simulink model "sbsb_srs_edit_7"  (R2023b)
settings: Solver=FixedStepDiscrete  StartTime=0.0  StopTime=100  FixedStep=0.001  RelTol=1e-3
libraries: Solver_SF x1
settings Model: DataTypeOverride=Double  MinMaxOverflowLogging=ForceOff  Creator=황수빈  LastModifiedBy=황수빈

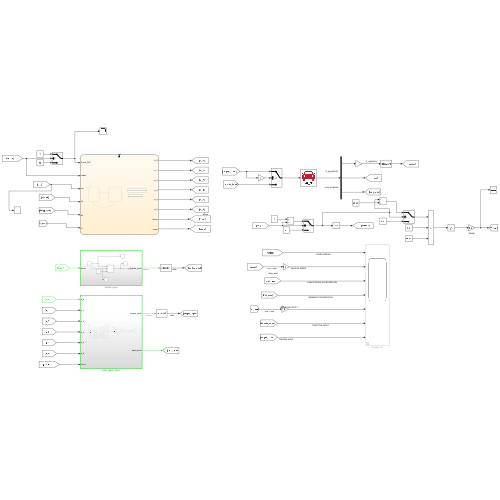
[thumbnail: Simulink's stored preview of the top-level diagram]
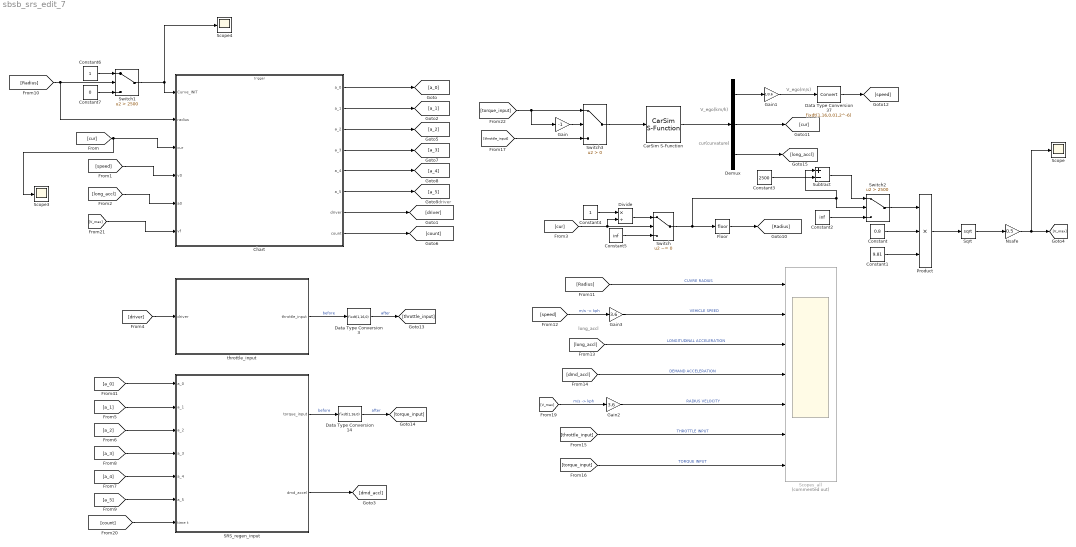
== system sbsb_srs_edit_7 ==
  note: driver
  note: long_accl
  note: V_ego(km/h)
  note: V_ego(m/s)
  note: cur(curvature)
  CarSim S-Function : Solver_SF/CarSim S-Function  Priority=1  SIMFILE=simfile.sim  Run_RTs=off  vs_state_ind=Run  StopMode_ind=Vehicle Model
  Chart : Stateflow chart  TreatAsAtomicUnit=on
  Constant : Constant  Value=0.8
  Constant1 : Constant  Value=9.81
  Constant2 : Constant  Value=inf
  Constant3 : Constant  Value=2500
  Constant4 : Constant
  Constant5 : Constant  Value=inf
  Constant6 : Constant
  Constant7 : Constant  Value=0
  Data Type Conversion14 : DataTypeConversion  OutDataTypeStr=fixdt(1,16,0)  RndMeth=Nearest  SaturateOnIntegerOverflow=off
  Data Type Conversion3 : DataTypeConversion  OutDataTypeStr=fixdt(1,16,0)  RndMeth=Nearest  SaturateOnIntegerOverflow=off
  Data Type Conversion37 : DataTypeConversion  OutDataTypeStr=fixdt(1,16,0.01,2^-6)  RndMeth=Simplest  SaturateOnIntegerOverflow=off
  Demux : Demux  Outputs=3
  Divide : Product  Inputs=*/
  Floor : Rounding
  Gain : Gain  Gain=-1
  Gain1 : Gain  Gain=1/3.6
  Gain2 : Gain  Gain=3.6
  Gain3 : Gain  Gain=3.6
  Nsafe : Gain  Gain=0.5
  Product : Product  Inputs=3
  SRS_regen_input : Subsystem  TreatAsAtomicUnit=on
  Scope : Scope
  Scope3 : Scope
  Scope4 : Scope
  Scopes_all : Scope  Commented=on  NumInputPorts=7
  Sqrt : Sqrt
  Subtract : Sum  Inputs=+-
  Switch : Switch  Criteria=u2 ~= 0  SaturateOnIntegerOverflow=off  InputSameDT=off
  Switch1 : Switch  Criteria=u2 > Threshold  Threshold=2500  SaturateOnIntegerOverflow=off  InputSameDT=off
  Switch2 : Switch  Criteria=u2 > Threshold  Threshold=2500  SaturateOnIntegerOverflow=off  InputSameDT=off
  Switch3 : Switch  Criteria=u2 > Threshold  SaturateOnIntegerOverflow=off  InputSameDT=off
  throttle_input : Subsystem  TreatAsAtomicUnit=on  SystemSampleTime=0.01
  wires:
  Chart/7(driver) -> [driver]
  [cur] -> Scope3/1, Chart/3(cur)
  [speed] -> Chart/4(v0)
  [long_accl] -> Chart/5(a0)
  Chart/1(a_0) -> [a_0]
  Chart/2(a_1) -> [a_1]
  Chart/3(a_2) -> [a_2]
  Chart/4(a_3) -> [a_3]
  Chart/5(a_4) -> [a_4]
  Chart/6(a_5) -> [a_5]
  Switch/1 -> Floor/1, Subtract/1, Switch2/2
  [cur] -> Switch/2, Divide/2
  Constant5/1 -> Switch/3
  Constant4/1 -> Divide/1
  Divide/1 -> Switch/1
  Gain1/1 -> Data Type Conversion37/1
  Demux/1 -> Gain1/1
  Demux/2 -> [cur]
  Data Type Conversion37/1 -> [speed]
  CarSim S-Function/1 -> Demux/1
  [driver] -> throttle_input/1(driver)
  Data Type Conversion3/1 -> [throttle_input]  "after"
  throttle_input/1(throttle_input) -> Data Type Conversion3/1  "before"
  SRS_regen_input/1(torque_input) -> Data Type Conversion14/1  "before"
  [a_2] -> SRS_regen_input/3(a_2)
  Data Type Conversion14/1 -> [torque_input]  "after"
  [a_0] -> SRS_regen_input/1(a_0)
  [a_3] -> SRS_regen_input/4(a_3)
  [a_5] -> SRS_regen_input/6(a_5)
  [Radius] -> Chart/2(radius), Switch1/2
  Constant6/1 -> Switch1/1
  Switch1/1 -> Scope4/1, Chart/1(Curve_INIT)
  Constant7/1 -> Switch1/3
  Demux/3 -> [long_accl]
  [Radius] -> Scopes_all/1  "CUVRE RADIUS"
  [speed] -> Gain3/1  "m/s -> kph"
  [long_accl] -> Scopes_all/3  "LONGITUDINAL ACCELERATION"
  [dmd_accl] -> Scopes_all/4  "DEMAND ACCELERATION"
  [V_max] -> Gain2/1  "m/s -> kph"
  [throttle_input] -> Scopes_all/6  "THROTTLE INPUT"
  SRS_regen_input/2(dmd_accel) -> [dmd_accl]
  Gain2/1 -> Scopes_all/5  "RADIUS VELOCITY"
  [a_1] -> SRS_regen_input/2(a_1)
  [a_4] -> SRS_regen_input/5(a_4)
  Chart/8(count) -> [count]
  [count] -> SRS_regen_input/7(time t)
  Sqrt/1 -> Nsafe/1
  Switch2/1 -> Product/1
  Constant/1 -> Product/2
  Constant1/1 -> Product/3
  Product/1 -> Sqrt/1
  Constant2/1 -> Switch2/3
  Nsafe/1 -> Scope/1, [V_max]
  [V_max] -> Chart/6(vf)
  Floor/1 -> [Radius]
  Switch3/1 -> CarSim S-Function/1
  [torque_input] -> Gain/1, Switch3/1
  [throttle_input] -> Switch3/3
  Gain/1 -> Switch3/2
  Constant3/1 -> Subtract/2
  Subtract/1 -> Switch2/1
  Gain3/1 -> Scopes_all/2  "VEHICLE SPEED"
  [torque_input] -> Scopes_all/7  "TORQUE INPUT"

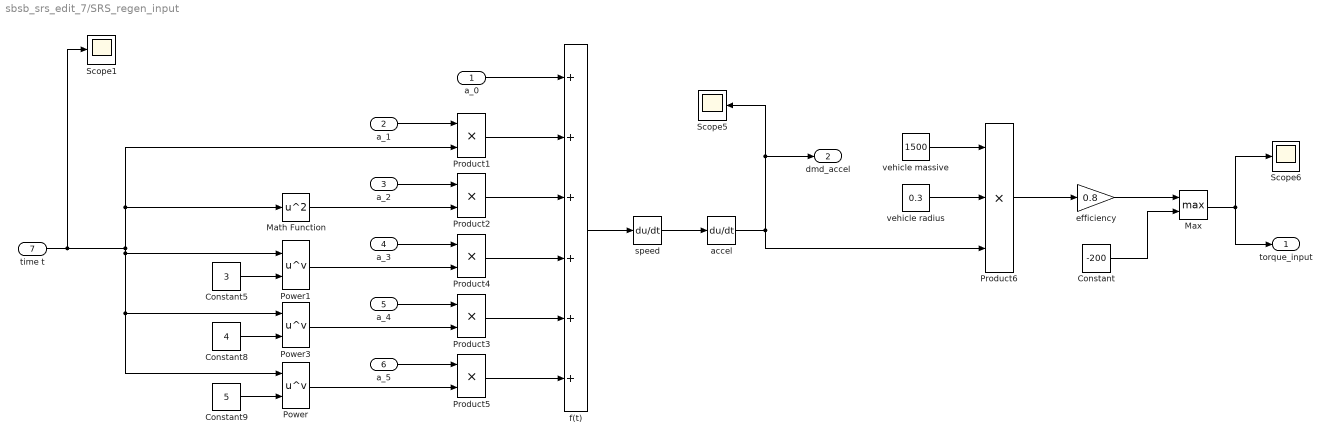
== system sbsb_srs_edit_7/SRS_regen_input ==
  a_0 : Inport
  a_1 : Inport  Port=2
  a_2 : Inport  Port=3
  a_3 : Inport  Port=4
  a_4 : Inport  Port=5
  a_5 : Inport  Port=6
  time t : Inport  Port=7
  Constant : Constant  Value=-200
  Constant5 : Constant  Value=3
  Constant8 : Constant  Value=4
  Constant9 : Constant  Value=5
  Math Function : Math  Operator=square
  Max : MinMax  Function=max  Inputs=2
  Power : Math  Operator=pow
  Power1 : Math  Operator=pow
  Power3 : Math  Operator=pow
  Product{1..5} (5 alike) : Product
  Product6 : Product  Inputs=3
  Scope1 : Scope
  Scope5 : Scope
  Scope6 : Scope
  accel : Derivative
  efficiency : Gain  Gain=0.8
  f(t) : Sum  Inputs=6
  speed : Derivative
  vehicle massive : Constant  Value=1500
  vehicle radius : Constant  Value=0.3
  torque_input : Outport
  dmd_accel : Outport  Port=2
  wires:
  a_0/1 -> f(t)/1
  f(t)/1 -> speed/1
  speed/1 -> accel/1
  accel/1 -> Product6/3, Scope5/1, dmd_accel/1
  time t/1 -> Power/1, Power3/1, Power1/1, Math Function/1, Product1/2, Scope1/1
  Constant9/1 -> Power/2
  Constant8/1 -> Power3/2
  Constant5/1 -> Power1/2
  a_1/1 -> Product1/1
  Product1/1 -> f(t)/2
  Product2/1 -> f(t)/3
  Product4/1 -> f(t)/4
  Product5/1 -> f(t)/6
  Product3/1 -> f(t)/5
  a_2/1 -> Product2/1
  a_3/1 -> Product4/1
  a_4/1 -> Product3/1
  a_5/1 -> Product5/1
  Power/1 -> Product5/2
  Power3/1 -> Product3/2
  Power1/1 -> Product4/2
  Math Function/1 -> Product2/2
  Product6/1 -> efficiency/1
  vehicle massive/1 -> Product6/1
  vehicle radius/1 -> Product6/2
  efficiency/1 -> Max/1
  Max/1 -> torque_input/1, Scope6/1
  Constant/1 -> Max/2

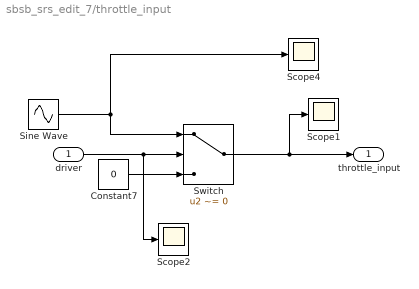
== system sbsb_srs_edit_7/throttle_input ==
  driver : Inport
  Constant7 : Constant  Value=0
  Scope1 : Scope
  Scope2 : Scope
  Scope4 : Scope
  Sine Wave : Sin  Amplitude=0.3
  Switch : Switch  Criteria=u2 ~= 0  Threshold=1  SaturateOnIntegerOverflow=off  InputSameDT=off
  throttle_input : Outport
  wires:
  driver/1 -> Scope2/1, Switch/2
  Switch/1 -> Scope1/1, throttle_input/1
  Constant7/1 -> Switch/3
  Sine Wave/1 -> Scope4/1, Switch/1

== stateflow chart sbsb_srs_edit_7/Chart ==
  state State1
    on entry:
    driver = 1;
    a_0 = 0;
    a_1 = 0;
    a_2 = 0;
    a_3 = 0;
    a_4 = 0;
    a_5 = 0;
    count = 0;
    distance = 0;
    time_final = 0;
    end
  state State4
    on entry:
    en : count = 0;
    if radius > 2500
    var_cal(radius, v0, vf);
    distance = distance;
    time_final = time_final;
    calculate(v0,a0,vf,distance,time_final);
    a_0 = a_0;
    a_1 = a_1;
    a_2 = a_2;
    a_3 = a_3;
    a_4 = a_4;
    a_5 = a_5;
    r_min = radius - 2500;
    end
    du: count = count + 1;
  (default) -> State1
  State1 -> State4 : [Curve_INIT == 1 ]
  State4 -> State1 : [radius == r_min || cur==0]
  data: v0 function_input; a0 function_input; vf function_input; a_0 function_output; a_1 function_output; a_2 function_output; a_3 function_output; a_4 function_output; a_5 function_output; distance function_input; time_final function_input; radius function_input; distance function_output; time_final function_output; v0 function_input; vf function_input; Curve_INIT input; radius input; cur input; v0 input; a0 input; a_0 output; a_1 output; a_2 output; a_3 output; a_4 output; a_5 output; driver output; r_min local; count output; vf input; distance local; time_final local
  events: entry input RISING_EDGE_EVENT
  function [a_0, a_1, a_2, a_3, a_4, a_5] =  calculate(v0, a0, vf, distance, time_final):
    | function [a_0, a_1, a_2, a_3, a_4, a_5] =  calculate(v0, a0, vf, distance, time_final)
    | 
    | % %curvature radius로 변환
    | % r = 1/c;
    | % maxradius = r - 2500; %최소곡률반지름
    | % 
    | % %% fd 이용한 목표 속도 계산 및 boundary conditions
    | % 
    | % %initial conditions at t = 0
    | % x0 = 0; v0 = v; a0 = a;
    | % 
    | % % 이차 방정식의 계수
    | % %radius = abs(sectioned_maxradius(initial));
    | % a = 1;
    | % b = 0.7493 * r;
    | % c = -127 * r * (0.2560 + 0.0037 * v0);
    | % 
    | % % 이차 방정식 풀이
    | % % v_fric2 = (-b ± sqrt(b^2 - 4ac)) / (2a)
    | % delta = b.^2 - 4 * a * c; % 판별식
    | % 
    | % % 판별식이 음수인 경우 복소수 해가 발생
    | % if any(delta < 0)
    | %     warning('Some values of delta are negative, which results in complex solutions.');
    | % end
    | % 
    | % %%final boundary conditions
    | % % 양수 해 계산
    | % v_fric2_positive = (-b + sqrt(delta)) / (2 * a);
    | % vf = v_fric2_positive;
    | % 
    | % %tf를 등가속도 공식으로 구하기
    | % tf = (vf - v0) / a0;
    | 
    | %% 5차 profiling %%
    | xf = distance; %아직 거리를 구하는 확정된 방법이 없으므로 등가속도 공식을 이용해서 구함
    | tf = time_final;
    | af = 0; %임의로 지정
    | 
    | A = [1, 0, 0, 0, 0, 0;
    |     0, 1, 0, 0, 0, 0;
    |     0, 0, 2, 0, 0, 0;
    |     1, tf, tf^2, tf^3, tf^4, tf^5;
    |     0, 1, 2*tf, 3*tf^2, 4*tf^3, 5*tf^4;
    |     0, 0, 2, 6*tf, 12*tf^2, 20*tf^3;];
    | 
    | B = [0; v0; a0; xf; vf; af;];
    | 
    | % coeffs = A/B;
    | % a_0 = coeffs(:,1);
    | % a_1 = coeffs(:,2);
    | % a_2 = coeffs(:,3);
    | % a_3 = coeffs(:,4);
    | % a_4 = coeffs(:,5);
    | % a_5 = coeffs(:,6);
    | 
    | % 연립 방정식 풀기 (A \ B 사용)
    | coeffs = A \ B;
    | 
    | % 계수 추출
    | a_0 = coeffs(1);
    | a_1 = coeffs(2);
    | a_2 = coeffs(3);
    | a_3 = coeffs(4);
    | a_4 = coeffs(5);
    | a_5 = coeffs(6);
  function [distance, time_final] = var_cal(radius, v0, vf):
    | function [distance, time_final] = var_cal(radius, v0, vf)
    |     % radius: 입력 값
    |     % v0: 초기 속도
    |     % vf: 최종 속도
    |     % distance: 조건에 따른 결과 값
    |     % tf: 계산된 시간 (distance / ((v0 + vf) / 2))
    | 
    |     % 조건에 따라 distance 설정
    |     if radius == 56
    |         distance = 1537.128;
    |     elseif radius == 108
    |         distance = 830.409;
    |     elseif radius == 220
    |         distance = 906.156;
    |             % 기본 값 설정
    |     else
    |             distance = NaN;  % 유효한 값이 없을 때 NaN 반환
    |     end
    |     
    |     % tf 계산 (distance가 NaN이 아니면 계산)
    |     if ~isnan(distance)
    |         time_final = distance / ((v0 + vf) / 2);  % 평균 속도를 사용하여 시간 계산
    |     else
    |         time_final = NaN;  % distance가 유효하지 않으면 tf도 NaN으로 설정
    |     end
    | end
